simulink model "pid_modelling"  (R2020b)
settings: Solver=VariableStepAuto  StartTime=0.0  StopTime=10.0  RelTol=1e-3
settings Model: Creator=amnessa  LastModifiedBy=amnessa

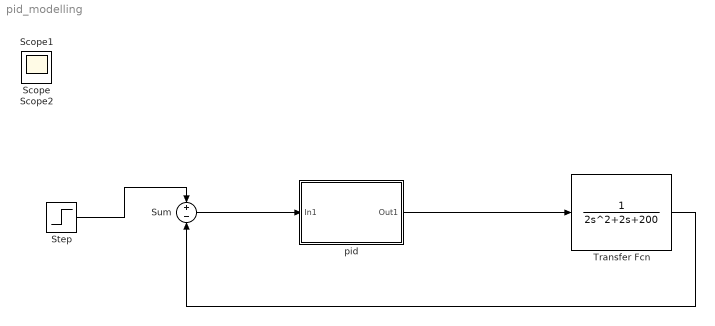
== system pid_modelling ==
  Step : Step  SampleTime=0
  Sum : Sum  Inputs=+-
  Transfer Fcn : TransferFcn  Denominator=[2 2 200]
  pid : Subsystem  mask{kp=1300, ki=700.0, kd=380.0}
      mask prompts: kp "proportional"; ki "integrational"; kd "derivational"
      mask DialogControl Container9 Prompt: Tab
  Scope : Scope
  Scope1 : Scope
  Scope2 : Scope
  wires:
  Transfer Fcn/1 -> Sum/2
  Step/1 -> Sum/1
  Sum/1 -> pid/1(In1)
  pid/1(Out1) -> Transfer Fcn/1

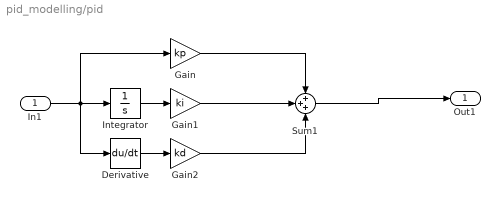
== system pid_modelling/pid ==
  In1 : Inport
  Derivative : Derivative
  Gain : Gain  Gain=kp
  Gain1 : Gain  Gain=ki
  Gain2 : Gain  Gain=kd
  Integrator : Integrator
  Sum1 : Sum  Inputs=+++
  Out1 : Outport
  wires:
  In1/1 -> Derivative/1, Gain/1, Integrator/1
  Gain2/1 -> Sum1/3
  Gain/1 -> Sum1/1
  Integrator/1 -> Gain1/1
  Gain1/1 -> Sum1/2
  Derivative/1 -> Gain2/1
  Sum1/1 -> Out1/1
